simulink model "ComparacionLineal_NoLineal"  (R2022b)
settings: Solver=VariableStepAuto  StartTime=0.0  StopTime=0.1  RelTol=1e-3
values from neighbouring files (symbols this model uses):
  A = argout.a    [linealizacion_hemsH8.m]
  B = argout.b    [linealizacion_hemsH8.m]
  C = argout.c    [linealizacion_hemsH8.m]
  D = -1900    [discretizacion.m]    (also in linealizacion_hemsH8.m = argout.d)
  g = 9.81    [hemsH8.m]
  m = i    [barrido_masas.m]    (also in hemsH8.m = 200)
undefined symbols (not defined in the file or in its folder): airgap, current, lev_nom
settings Model: Creator=ramuj  LastModifiedBy=aceao

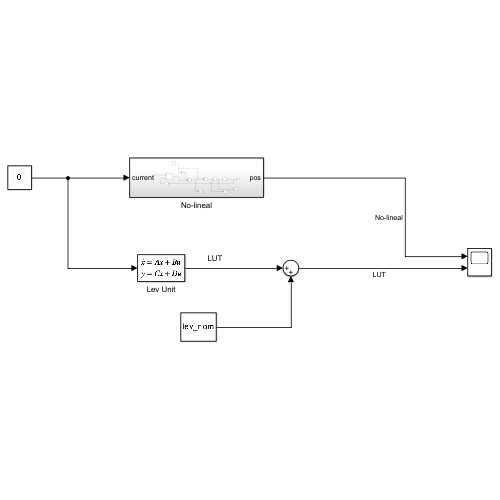
[thumbnail: Simulink's stored preview of the top-level diagram]
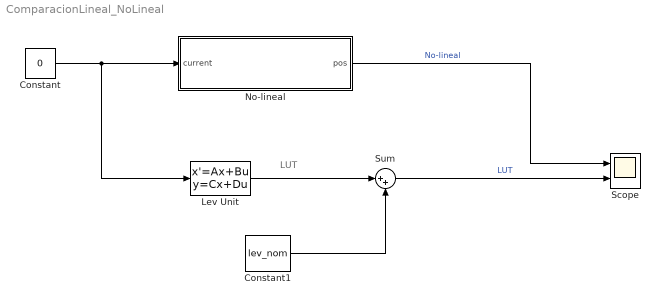
== system ComparacionLineal_NoLineal ==
  note: LUT
  Constant : Constant  Value=0
  Constant1 : Constant  Value=lev_nom
  Lev Unit : StateSpace  A=A  B=B  C=C  D=D  InitialCondition=[1e-3 0]  ParameterTunability=Unconstrained
  No-lineal : Subsystem
  Scope : Scope  NumInputPorts=2
  Sum : Sum  Inputs=|++
  wires:
  Lev Unit/1 -> Sum/1
  Constant1/1 -> Sum/2
  Constant/1 -> Lev Unit/1, No-lineal/1(current)
  No-lineal/1(pos) -> Scope/1  "No-lineal"
  Sum/1 -> Scope/2  "LUT"

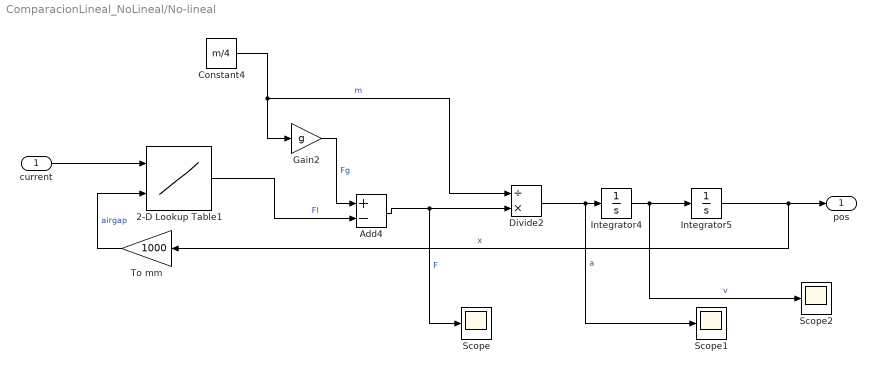
== system ComparacionLineal_NoLineal/No-lineal ==
  current : Inport
  2-D Lookup Table1 : Lookup_n-D  BreakpointsForDimension1=current(1,:)  BreakpointsForDimension2=airgap(:,1)  Table=force'  InternalRulePriority=Speed  RndMeth=Simplest
      settings: InputPortMap=u0,u1
  Add4 : Sum  Inputs=+-
  Constant4 : Constant  Value=m/4
  Divide2 : Product  Inputs=/*
  Gain2 : Gain  Gain=g
  Integrator4 : Integrator
  Integrator5 : Integrator  InitialCondition=lev_nom+1e-3
  Scope : Scope
  Scope1 : Scope
  Scope2 : Scope
  To mm : Gain  Gain=1000
  pos : Outport
  wires:
  Integrator5/1 -> pos/1, To mm/1  "x"
  Constant4/1 -> Gain2/1, Divide2/1  "m"
  Divide2/1 -> Scope1/1, Integrator4/1  "a"
  To mm/1 -> 2-D Lookup Table1/2  "airgap"
  Integrator4/1 -> Scope2/1, Integrator5/1  "v"
  Add4/1 -> Scope/1, Divide2/2  "F"
  current/1 -> 2-D Lookup Table1/1
  2-D Lookup Table1/1 -> Add4/2  "Fl"
  Gain2/1 -> Add4/1  "Fg"
